simulink model "Tega"  (R2023b)
settings: Solver=VariableStepAuto  StartTime=0.0  StopTime=10.0  RelTol=1e-3
libraries: spsSeriesRLCBranchLib x4, spsCurrentMeasurementLib x1, spsDiodeLib x1, spsIGBTDiodeLib x1, spsPVArrayLib x1, spsPWMGeneratorDCDCLib x1, spsVoltageMeasurementLib x1, sps_lib x1
settings Model: Creator=HP  LastModifiedBy=HP

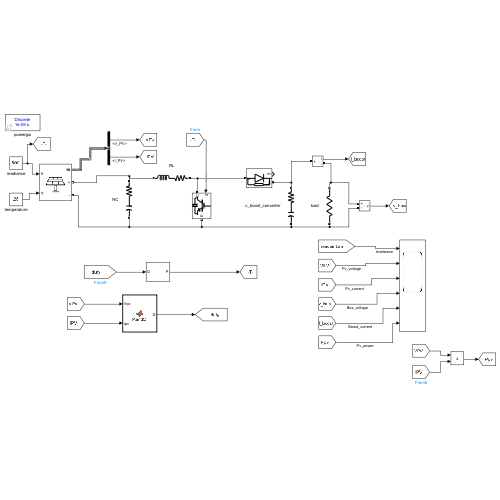
[thumbnail: Simulink's stored preview of the top-level diagram]
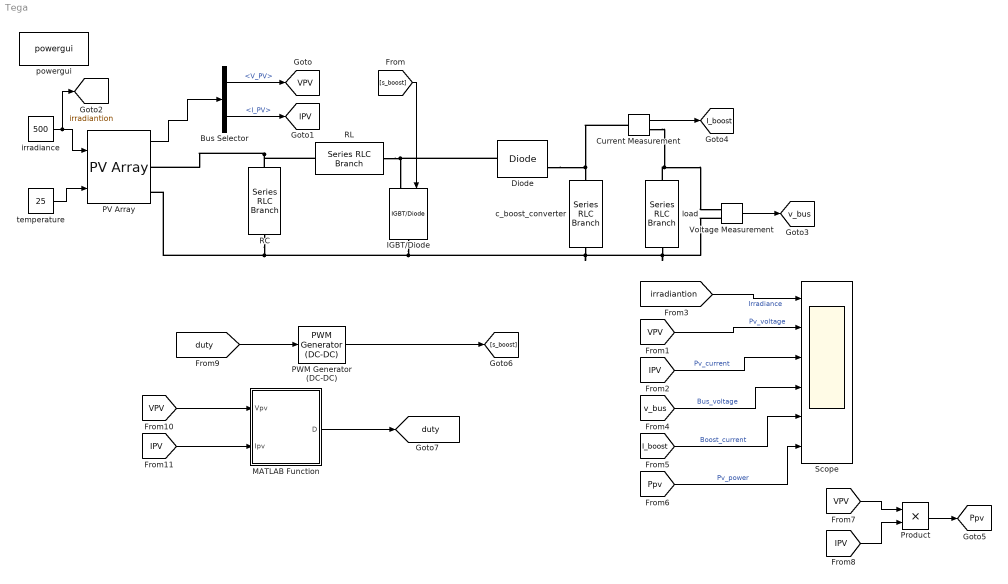
== system Tega ==
  Bus Selector : BusSelector  OutputSignals=V_PV,I_PV
  Current Measurement : spsCurrentMeasurementLib/Current Measurement  PhasorSimulation=off  OutputType=Complex  PSBequivalent=0
  Diode : spsDiodeLib/Diode  Ron=0.001  Lon=0  Vf=0.8  IC=0  UseSnubber=0  Rs=500  Cs=250e-9  Measurements=on
  IGBT/Diode : spsIGBTDiodeLib/IGBT//Diode  Ron=1e-3  Rs=1e5  Cs=inf  Measurements=off
  MATLAB Function : MATLAB Function  TreatAsAtomicUnit=on
  PV Array : spsPVArrayLib/PV Array  Npar=6  Nser=2  PlotType=array @ 1000 W/m2 & specified temperatures  S_vec="[ 1000  500  100 ]"  Temp_C_vec="[ 45 25  ]"  ModuleName=User-defined  PlotWhenSelected=off  Pm=380.16  Ncell=72  Voc=48.7  Isc=9.98  Vm=39.6  Im=9.6  beta_Voc_pc=-0.32  alpha_Isc_pc=0.05  beta_Voc=-0.15584  alpha_Isc=0.00499  IL=10.0548  I0=7.7106e-11  nI=1.0287  Rsh=2826.5806  Rs=0.35496  RobustModel=off  RobustCellTemperature=313.3991  BAL=on  Tc=1e-6  Tfilter=5e-5
  PWM Generator (DC-DC) : spsPWMGeneratorDCDCLib/PWM Generator (DC-DC)  Fsw=5000  Ts=10e-6
  Product : Product
  RC : spsSeriesRLCBranchLib/Series RLC Branch  LConnTagsString=__new0  RConnTagsString=__new0  BranchType=RC  Resistance=1e-4  Inductance=1e-3  SetiL0=off  InitialCurrent=0  Capacitance=100e-6  Setx0=off  InitialVoltage=0  Measurements=None
  RL : spsSeriesRLCBranchLib/Series RLC Branch  LConnTagsString=__new0  RConnTagsString=__new0  BranchType=RL  Resistance=0.1  Inductance=5e-3  SetiL0=off  InitialCurrent=0  Capacitance=100e-6  Setx0=off  InitialVoltage=0  Measurements=None
  Scope : Scope  NumInputPorts=6
  Voltage Measurement : spsVoltageMeasurementLib/Voltage Measurement  PhasorSimulation=off  OutputType=Complex  PSBequivalent=0
  c_boost_converter : spsSeriesRLCBranchLib/Series RLC Branch  LConnTagsString=__new0  RConnTagsString=__new0  BranchType=RC  Resistance=1e-4  Inductance=1e-3  SetiL0=off  InitialCurrent=0  Capacitance=3300e-6  Setx0=off  InitialVoltage=0  Measurements=None
  irradiance : Constant  Value=500
  load : spsSeriesRLCBranchLib/Series RLC Branch  LConnTagsString=__new0  RConnTagsString=__new0  BranchType=R  Resistance=10  Inductance=1e-3  SetiL0=off  InitialCurrent=0  Capacitance=3300e-6  Setx0=off  InitialVoltage=0  Measurements=None
  powergui : sps_lib/powergui  Priority=1  SimulationMode=Discrete  SampleTime=1e-05  frequency=60  Iterations=50  frequencyindice=0  Pbase=100e6  ErrMax=1e-4  UnitsV=kV  UnitsW=MW  buscounter=0  FunctionMessages=off  echomessages=off  EnableUseOfTLC=off  CurrentSourceSwitches=off  DisableSnubberDevices=off  DisableRonSwitches=off  DisableVfSwitches=off  DisplayEquations=off  AutomaticDiscreteSolvers=off  SolverType=Tustin/Backward Euler (TBE)  Interpol=off  ExternalGateDelay=off  methode=off  Ts=100  x0status=blocks  SPID=on  SwTol=0  HookPort=off  NonlinearTolerance=1e-4  nMaxIteration=100  ContinueOnMaxIteration=off  RestoreLinks=warning  ResistiveCurrentMeasurement=off  Frange=[0:2:500]  Ylog=off  Xlog=on  ShowGrid=off  save=off  variable=ZData  structure=0  ZoomFFT=off  StartTime=0.0  cycles=1  DisplayStyle=1  fundamental=60  FreqAxis=off  MaxFrequency=1000  frequencyindicesteady=1  RmsSteady=1  display=off
  temperature : Constant  Value=25
  tag scope: IPV=global, I_boost=global, Ppv=global, VPV=global, duty=global, irradiantion=global, v_bus=global
  wires:
  PV Array/1 -> Bus Selector/1
  Bus Selector/1 -> [VPV]  "<V_PV>"
  Bus Selector/2 -> [IPV]  "<I_PV>"
  temperature/1 -> PV Array/2
  irradiance/1 -> [irradiantion], PV Array/1
  [s_boost] -> IGBT/Diode/1
  Voltage Measurement/1 -> [v_bus]
  Current Measurement/1 -> [I_boost]
  [irradiantion] -> Scope/1  "Irradiance"
  [VPV] -> Scope/2  "Pv_voltage"
  [IPV] -> Scope/3  "Pv_current"
  [v_bus] -> Scope/4  "Bus_voltage"
  [I_boost] -> Scope/5  "Boost_current"
  [Ppv] -> Scope/6  "Pv_power"
  Product/1 -> [Ppv]
  [VPV] -> Product/1
  [IPV] -> Product/2
  PWM Generator (DC-DC)/1 -> [s_boost]
  [duty] -> PWM Generator (DC-DC)/1
  [VPV] -> MATLAB Function/1(Vpv)
  [IPV] -> MATLAB Function/2(Ipv)
  MATLAB Function/1(D) -> [duty]
  connections:
  RC/LConn1 -- RL/RConn1 -- PV Array/RConn1
  RC/RConn1 -- Voltage Measurement/LConn2 -- load/RConn1 -- c_boost_converter/RConn1 -- IGBT/Diode/RConn1 -- PV Array/RConn2
  RL/LConn1 -- Diode/LConn1 -- IGBT/Diode/LConn1
  Diode/RConn1 -- Current Measurement/LConn1 -- c_boost_converter/LConn1
  load/LConn1 -- Current Measurement/RConn1 -- Voltage Measurement/LConn1

== matlab function Tega/MATLAB Function ==
  data: Vpv input; D output; Ipv input
function D = PandO(Vpv, Ipv)

persistent Dprev Pprev Vprev

if isempty(Dprev)
    Dprev = 0.7;
    Vprev = 190;
    Pprev = 2000;
end

deltaD = 125e-6;

%calculate measured aerray power
Ppv = Vpv*Ipv; 

%Increase or decrease duty cycle based on conditions
if (Ppv-Pprev) ~= 0
    if (Ppv-Pprev) > 0
        if (Vpv-Vprev) > 0
            D = Dprev - deltaD;
        else
            D = Dprev + deltaD;
        end
    else
        if (Vpv-Vprev) > 0
            D = Dprev + deltaD;
        else
            D = Dprev - deltaD;
        end
    end
else
    D =Dprev;
end

%Update internal values
Dprev = D;
Vprev = Vpv;
Pprev = Ppv;
